simulink model "PID"  (R2017b)
settings: Solver=VariableStepAuto  StartTime=0.0  StopTime=10.0  RelTol=1e-3
libraries: simulink x3
settings Model: Creator=Пользователь  LastModifiedBy=Пользователь

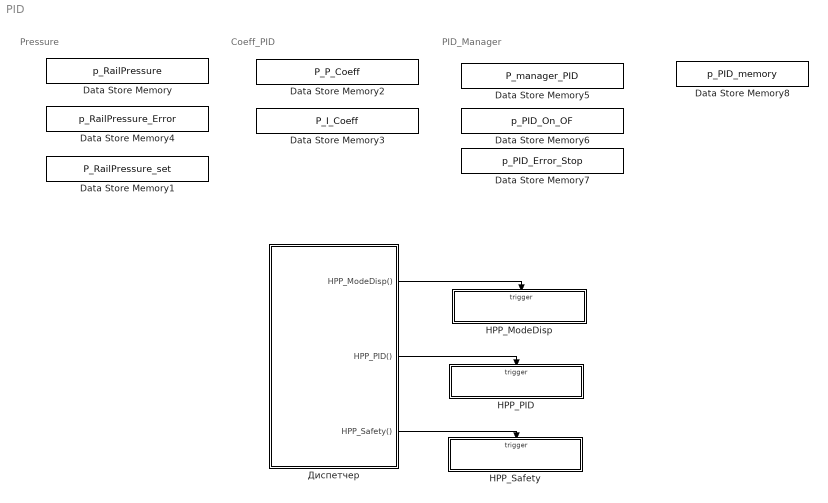
== system PID ==
  note: PID_Manager
  note: Coeff_PID
  note: Pressure
  Data Store Memory : DataStoreMemory  DataStoreName=p_RailPressure  ReadBeforeWriteMsg=warning  WriteAfterWriteMsg=warning  WriteAfterReadMsg=warning  ShowAdditionalParam=off  OutMin=0  OutMax=4500  OutDataTypeStr=fixdt(0,32,19)
  Data Store Memory1 : DataStoreMemory  DataStoreName=P_RailPressure_set  ReadBeforeWriteMsg=warning  WriteAfterWriteMsg=warning  WriteAfterReadMsg=warning  ShowAdditionalParam=off  OutMin=0  OutMax=4500  OutDataTypeStr=fixdt(0,32,19)
  Data Store Memory2 : DataStoreMemory  DataStoreName=P_P_Coeff  ReadBeforeWriteMsg=warning  WriteAfterWriteMsg=warning  WriteAfterReadMsg=warning  ShowAdditionalParam=off  OutMin=-10  OutMax=10  OutDataTypeStr=fixdt(1,32,27)
  Data Store Memory3 : DataStoreMemory  DataStoreName=P_I_Coeff  ReadBeforeWriteMsg=warning  WriteAfterWriteMsg=warning  WriteAfterReadMsg=warning  ShowAdditionalParam=off  OutMin=-10  OutMax=10  OutDataTypeStr=fixdt(1,32,27)
  Data Store Memory4 : DataStoreMemory  DataStoreName=p_RailPressure_Error  ReadBeforeWriteMsg=warning  WriteAfterWriteMsg=warning  WriteAfterReadMsg=warning  ShowAdditionalParam=off  OutMin=0  OutMax=4500  OutDataTypeStr=fixdt(1,32,18)
  Data Store Memory5 : DataStoreMemory  DataStoreName=P_manager_PID  ReadBeforeWriteMsg=warning  WriteAfterWriteMsg=warning  WriteAfterReadMsg=warning  ShowAdditionalParam=off  OutMin=0  OutMax=1  OutDataTypeStr=fixdt(0,32,31)
  Data Store Memory6 : DataStoreMemory  DataStoreName=p_PID_On_OF  ReadBeforeWriteMsg=warning  WriteAfterWriteMsg=warning  WriteAfterReadMsg=warning  ShowAdditionalParam=off  OutMin=0  OutMax=1  OutDataTypeStr=fixdt(0,32,31)
  Data Store Memory7 : DataStoreMemory  DataStoreName=p_PID_Error_Stop  ReadBeforeWriteMsg=warning  WriteAfterWriteMsg=warning  WriteAfterReadMsg=warning  ShowAdditionalParam=off  OutMin=0  OutMax=1  OutDataTypeStr=fixdt(0,32,31)
  Data Store Memory8 : DataStoreMemory  DataStoreName=p_PID_memory  ReadBeforeWriteMsg=warning  WriteAfterWriteMsg=warning  WriteAfterReadMsg=warning  ShowAdditionalParam=off  OutMin=0  OutMax=100  OutDataTypeStr=fixdt(1,32,24)
  HPP_ModeDisp : Subsystem
  HPP_PID : Subsystem
  "HPP_Safety " : Subsystem
  Диспетчер : Stateflow chart  TreatAsAtomicUnit=on
  wires:
  Диспетчер/2(HPP_PID()) -> HPP_PID/Trigger
  Диспетчер/1(HPP_ModeDisp()) -> HPP_ModeDisp/Trigger
  Диспетчер/3(HPP_Safety()) -> "HPP_Safety "/Trigger

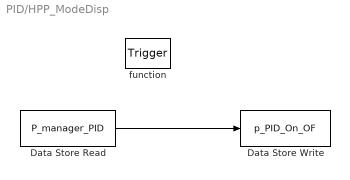
== system PID/HPP_ModeDisp ==
  function : TriggerPort  TriggerType=function-call  VariantControl=(inherit)
  Data Store Read : DataStoreRead  DataStoreName=P_manager_PID
  Data Store Write : DataStoreWrite  DataStoreName=p_PID_On_OF
  wires:
  Data Store Read/1 -> Data Store Write/1

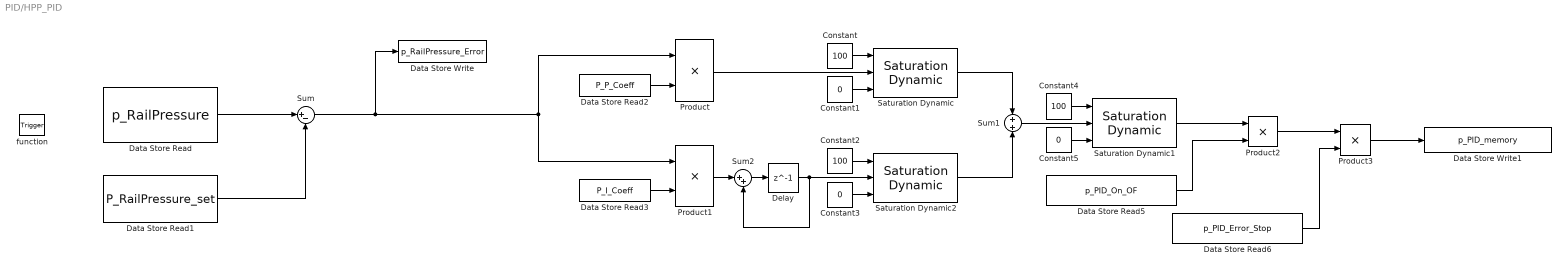
== system PID/HPP_PID ==
  function : TriggerPort  TriggerType=function-call  VariantControl=(inherit)
  Constant : Constant  Value=100
  Constant1 : Constant  Value=0
  Constant2 : Constant  Value=100
  Constant3 : Constant  Value=0
  Constant4 : Constant  Value=100
  Constant5 : Constant  Value=0
  Data Store Read : DataStoreRead  DataStoreName=p_RailPressure
  Data Store Read1 : DataStoreRead  DataStoreName=P_RailPressure_set  DataStoreElements=P_RailPressure_set
  Data Store Read2 : DataStoreRead  DataStoreName=P_P_Coeff
  Data Store Read3 : DataStoreRead  DataStoreName=P_I_Coeff
  Data Store Read5 : DataStoreRead  DataStoreName=p_PID_On_OF
  Data Store Read6 : DataStoreRead  DataStoreName=p_PID_Error_Stop
  Data Store Write : DataStoreWrite  DataStoreName=p_RailPressure_Error
  Data Store Write1 : DataStoreWrite  DataStoreName=p_PID_memory
  Delay : Delay  DelayLength=1  InitialCondition=0
  Product{,1..3} (4 alike) : Product
  Saturation Dynamic : simulink/Discontinuities/Saturation Dynamic  OutMin=[]  OutMax=[]  OutDataTypeStr=Inherit: Same as second input  OutDataType=fixdt(1, 16)  OutScaling=2^-10  DoSatur=off
  Saturation Dynamic1 : simulink/Discontinuities/Saturation Dynamic  OutMin=[]  OutMax=[]  OutDataTypeStr=Inherit: Same as second input  OutDataType=fixdt(1, 16)  OutScaling=2^-10  DoSatur=off
  Saturation Dynamic2 : simulink/Discontinuities/Saturation Dynamic  OutMin=[]  OutMax=[]  OutDataTypeStr=Inherit: Same as second input  OutDataType=fixdt(1, 16)  OutScaling=2^-10  DoSatur=off
  Sum : Sum  Inputs=|+-
  Sum1 : Sum
  Sum2 : Sum  Inputs=|++
  wires:
  Data Store Read1/1 -> Sum/2
  Sum1/1 -> Saturation Dynamic1/2
  Data Store Read/1 -> Sum/1
  Data Store Read2/1 -> Product/2
  Product/1 -> Saturation Dynamic/2
  Constant1/1 -> Saturation Dynamic/3
  Constant/1 -> Saturation Dynamic/1
  Saturation Dynamic1/1 -> Product2/1
  Saturation Dynamic/1 -> Sum1/1
  Data Store Read3/1 -> Product1/2
  Product1/1 -> Sum2/1
  Sum2/1 -> Delay/1
  Delay/1 -> Saturation Dynamic2/2, Sum2/2
  Constant2/1 -> Saturation Dynamic2/1
  Constant3/1 -> Saturation Dynamic2/3
  Constant4/1 -> Saturation Dynamic1/1
  Constant5/1 -> Saturation Dynamic1/3
  Saturation Dynamic2/1 -> Sum1/2
  Sum/1 -> Product1/1, Product/1, Data Store Write/1
  Data Store Read5/1 -> Product2/2
  Product2/1 -> Product3/1
  Data Store Read6/1 -> Product3/2
  Product3/1 -> Data Store Write1/1

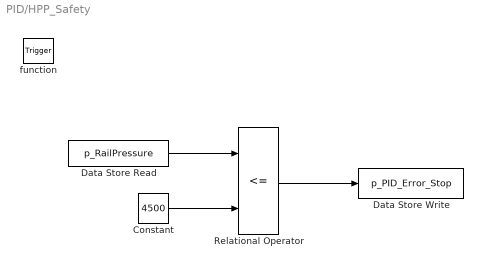
== system PID/HPP_Safety  ==
  function : TriggerPort  TriggerType=function-call  VariantControl=(inherit)
  Constant : Constant  Value=4500  OutDataTypeStr=uint32
  Data Store Read : DataStoreRead  DataStoreName=p_RailPressure
  Data Store Write : DataStoreWrite  DataStoreName=p_PID_Error_Stop
  Relational Operator : RelationalOperator  Operator=<=  OutDataTypeStr=boolean  RndMeth=Simplest
  wires:
  Data Store Read/1 -> Relational Operator/1
  Constant/1 -> Relational Operator/2
  Relational Operator/1 -> Data Store Write/1

== stateflow chart PID/Диспетчер ==
  (junction 123) -> (junction 124) : {HPP_ModeDisp;
      | HPP_PID;
      | HPP_Safety;
      | }
  events: HPP_ModeDisp output FUNCTION_CALL_EVENT; HPP_PID output FUNCTION_CALL_EVENT; HPP_Safety output FUNCTION_CALL_EVENT
